simulink model "Simu_3"  (R2013a)
settings: Solver=ode45  StartTime=0.0  StopTime=3  RelTol=1e-3
libraries: fl_lib x5, elec_lib x4, nesl_utility x3
settings Model: Creator=Polotto  LastModifiedBy=Polotto

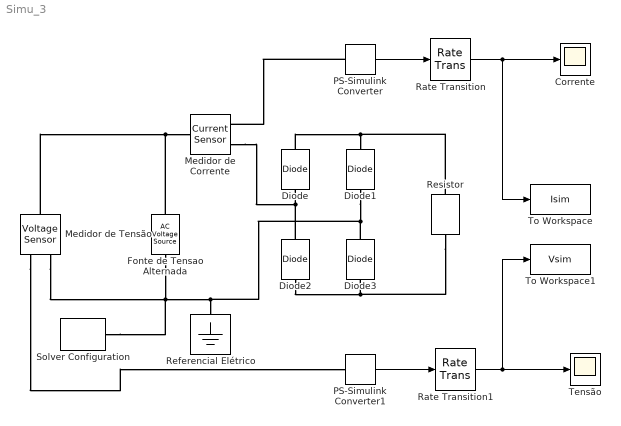
== system Simu_3 ==
  Corrente : Scope
      settings: YMin=-175  YMax=175
  Diode{,1..3} (4 alike) : elec_lib/Semiconductor Devices/Diode  ModelType=1  Vf=0.6 V  Ron=0.3 Ohm  Goff=1e-8 S  Rz=0.3 Ohm  Vz=50 V  C_PWL=5 pF  prmExp=1  I12=[ 0.0137 0.545 ] A  V12=[ 0.6 0.7 ] V  I1=0.0137 A  V1=0.6 V  RS=0.01 Ohm  IS=1e-12 A  Tmeas=25 C  ec=1  BV=Inf V  C_param=1  CJ0=5 pF  VJ=1 V  Mgrad=0.5  Vvec=[ 0.1 10 100 ] V  Cvec=[ 3.5 1 0.4 ] pF  FC=0.5  Q_param=1  Irrm=-7.15 A  iF=4 A  didt=-750 A/us  trr=115 ns  TT=50 ns  tau=100 ns  T_param=1  IS_T2=1.25e-7 A  I1_T2=0.245 A  V1_T2=0.5 V  Tmeas2=125 C  EG_param=1  EG=1.11 eV  XTI_param=1  XTI=3  dBVdT=0 V/K  Tdevice=25 C  LocalVarLogging=[]  Rth=[ 0 10 ] K/W  thermal_mass_parameterization=1  thermal_mass=[ 0 1 ] J/K  thermal_time_constant=[ 0 10 ] s  thermal_mass_initial_temperatures=[ 25 25 ] C
  Fonte de Tensao Alternada : fl_lib/Electrical/Electrical Sources/AC Voltage Source  amp=127*sqrt(2) V  shift=0 deg  frequency=60 Hz  omega=0 rad/s  i_Log=off  v_Log=off  LocalVarNames=|i|v  LocalVarDescs=|i|v  LocalVarLogging=[0 0]
  Medidor de Corrente : fl_lib/Electrical/Electrical Sensors/Current Sensor  i1_Log=off  v1_Log=off  LocalVarNames=|i1|v1  LocalVarDescs=|i1|v1  LocalVarLogging=[0 0]
  Medidor de Tensão : fl_lib/Electrical/Electrical Sensors/Voltage Sensor  i1_Log=off  v1_Log=off  LocalVarNames=|i1|v1  LocalVarDescs=|i1|v1  LocalVarLogging=[0 0]
  PS-Simulink Converter : nesl_utility/PS-Simulink Converter  PhysicalDomain=network_engine_domain  SubClassName=ps_output  LeftPortType=input  RightPortType=output  PseudoPeriodic=off  Frequencies=[]  Unit=1  AffineConversion=off
  PS-Simulink Converter1 : nesl_utility/PS-Simulink Converter  PhysicalDomain=network_engine_domain  SubClassName=ps_output  LeftPortType=input  RightPortType=output  PseudoPeriodic=off  Frequencies=[]  Unit=1  AffineConversion=off
  Rate Transition : RateTransition  OutPortSampleTimeOpt=Multiple of input port sample time  OutPortSampleTimeMultiple=0.2  OutPortSampleTime=0.1
  Rate Transition1 : RateTransition  OutPortSampleTimeOpt=Multiple of input port sample time  OutPortSampleTimeMultiple=0.2  OutPortSampleTime=0.1
  Referencial Elétrico : fl_lib/Electrical/Electrical Elements/Electrical Reference  i_Log=off  LocalVarNames=|i  LocalVarDescs=|i  LocalVarLogging=0
  Resistor : fl_lib/Electrical/Electrical Elements/Resistor  R=10 Ohm  i_Log=off  v_Log=off  LocalVarNames=|i|v  LocalVarDescs=|i|v  LocalVarLogging=[0 0]
  Solver Configuration : nesl_utility/Solver Configuration  PhysicalDomain=network_engine_domain  SubClassName=solver  LeftPortType=input  RightPortType=generic  Accelerate=off  Tones=[]  Harmonics=[]  SimulateNoise=off  Profile=off  UseLocalSampling=off  EnableSwitchedLinearOptims=on  FrequencyDomain=off  UseCCode=off  UseNewInitialization=off  DoDC=off  ResidualTolerance=1e-09  UseLocalSolver=on  LocalSolverChoice=NE_BACKWARD_EULER_ADVANCER  LocalSolverSampleTime=0.0001  DoFixedCost=on  MaxNonlinIter=5  MaxModeIter=2  LinearAlgebra=Sparse  DelaysMemoryBudget=1024
  Tensão : Scope
      settings: YMin=-175  YMax=175
  To Workspace : ToWorkspace  VariableName=Isim  SampleTime=-1  SaveFormat=Structure With Time
  To Workspace1 : ToWorkspace  VariableName=Vsim  SampleTime=-1  SaveFormat=Structure With Time
  wires:
  PS-Simulink Converter/1 -> Rate Transition/1
  PS-Simulink Converter1/1 -> Rate Transition1/1
  Rate Transition/1 -> To Workspace/1, Corrente/1
  Rate Transition1/1 -> To Workspace1/1, Tensão/1
  connections:
  Medidor de Tensão/RConn2 -- Fonte de Tensao Alternada/RConn1 -- Solver Configuration/RConn1 -- Diode1/LConn1 -- Diode3/RConn1 -- Referencial Elétrico/LConn1
  Medidor de Tensão/LConn1 -- Fonte de Tensao Alternada/LConn1 -- Medidor de Corrente/LConn1
  PS-Simulink Converter/LConn1 -- Medidor de Corrente/RConn1
  Medidor de Tensão/RConn1 -- PS-Simulink Converter1/LConn1
  Diode2/LConn1 -- Resistor/RConn1 -- Diode3/LConn1
  Diode/RConn1 -- Resistor/LConn1 -- Diode1/RConn1
  Medidor de Corrente/RConn2 -- Diode2/RConn1 -- Diode/LConn1
